simulink model "cruise_control_aberta"  (R2022b)
settings: Solver=FixedStepAuto  StartTime=0.0  StopTime=100  FixedStep=1e-3  RelTol=1e-3
values from neighbouring files (symbols this model uses):
  b = f/v(end)    [identificarCruiseControl.m]
  m = -b * t(1000) / log(1 - (b/f) * v(1000))    [identificarCruiseControl.m]
undefined symbols (not defined in the file or in its folder): d
settings Model: Creator=mmaximo  LastModifiedBy=danie
settings SolverCC: AlgebraicLoopSolver=TrustRegion
settings DebuggingCC: UnconnectedInputMsg=warning  UnconnectedOutputMsg=warning  UnconnectedLineMsg=warning  SFMachineParentedDataDiag=warning
settings ModelReferenceCC: EnableRefExpFcnMdlSchedulingChecks=on
settings RTWCC: DLArmComputeVersion=19.05

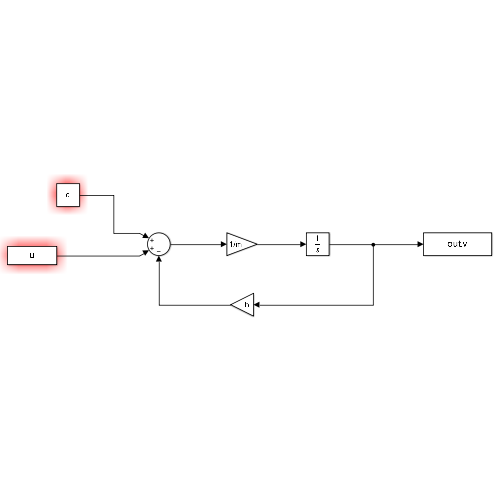
[thumbnail: Simulink's stored preview of the top-level diagram]
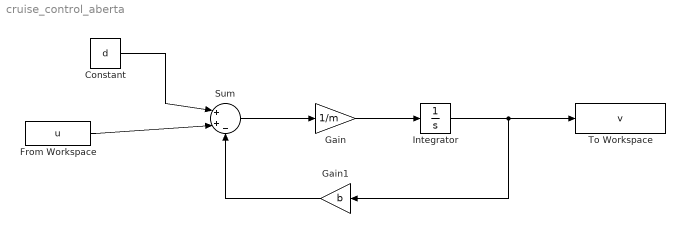
== system cruise_control_aberta ==
  Constant : Constant  Value=d
  From Workspace : FromWorkspace  VariableName=u
  Gain : Gain  Gain=1/m
  Gain1 : Gain  Gain=b
  Integrator : Integrator
  Sum : Sum  Inputs=|++-
  To Workspace : ToWorkspace  VariableName=v  SaveFormat=Structure With Time  SampleTime=-1
  wires:
  From Workspace/1 -> Sum/2
  Gain/1 -> Integrator/1
  Integrator/1 -> Gain1/1, To Workspace/1
  Gain1/1 -> Sum/3
  Sum/1 -> Gain/1
  Constant/1 -> Sum/1
